simulink model "a04_standartregelkreis_part_b"  (R2018a)
settings: Solver=VariableStepAuto  StartTime=0.0  StopTime=10.0  RelTol=1e-3
settings Model: Creator=oleksandra  LastModifiedBy=oleksandra

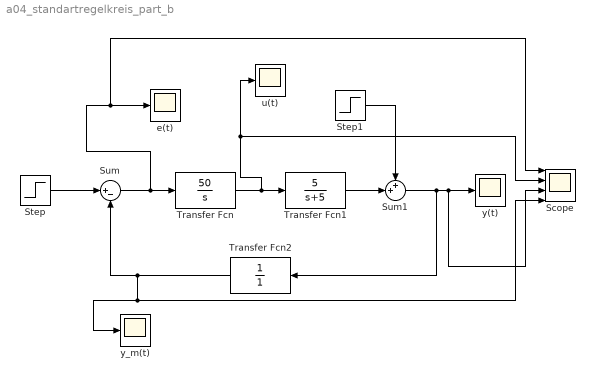
== system a04_standartregelkreis_part_b ==
  Scope : Scope  NumInputPorts=4
  Step : Step  Time=0  After=5  SampleTime=0
  Step1 : Step  Time=2  After=6  SampleTime=0
  Sum : Sum  Inputs=|+-
  Sum1 : Sum  Inputs=++|
  Transfer Fcn : TransferFcn  Numerator=[0 50]  Denominator=[1 0 ]
  Transfer Fcn1 : TransferFcn  Numerator=[0 5]  Denominator=[1 5]
  Transfer Fcn2 : TransferFcn  Denominator=[1]
  e(t) : Scope
  u(t) : Scope
  y(t) : Scope
  y_m(t) : Scope
  wires:
  Step/1 -> Sum/1
  Sum/1 -> Scope/1, e(t)/1, Transfer Fcn/1
  Transfer Fcn/1 -> Scope/2, u(t)/1, Transfer Fcn1/1
  Transfer Fcn1/1 -> Sum1/2
  Step1/1 -> Sum1/1
  Sum1/1 -> Transfer Fcn2/1, Scope/3, y(t)/1
  Transfer Fcn2/1 -> Scope/4, y_m(t)/1, Sum/2
